simulink model "XLS_detumbling"  (R2017b)
settings: Solver=FixedStepAuto  StartTime=0.0  StopTime=25000  FixedStep=0.1  RelTol=1e-3  EnableMultiTasking=on
values from neighbouring files (symbols this model uses):
  attitude_0 = [0,0,0]    [ga_detumbling.m]    (also in ga_detumbling_fit.m = [0.0524,-0.0349,0.0175]; ga_pid.m; ga_pid_fit.m; ga_pid_test.m)
  attitude_rate_0 = [0,6.7e-05,0.0041]    [ga_detumbling.m]    (also in ga_detumbling_fit.m = [0.0873,-0.0873,-0.0873]; ga_pid.m; ga_pid_fit.m; ga_pid_test.m)
  dp = x(2)    [ga_detumbling.m]    (also in ga_detumbling_fit.m = d(2); ga_pid.m = x(4); ga_pid_fit.m = d(4); ga_pid_test.m = x(4))
  dr = x(1)    [ga_detumbling.m]    (also in ga_detumbling_fit.m = d(1); ga_pid.m = x(2); ga_pid_fit.m = d(2); ga_pid_test.m = x(2))
  dy = x(3)    [ga_detumbling.m]    (also in ga_detumbling_fit.m = d(3); ga_pid.m = x(6); ga_pid_fit.m = d(6); ga_pid_test.m = x(6))
libraries: simulink_extras x5, aerolibanim x1, sharedutil x1
CloseFcn:
  | rtwprivate ssgencode ModelCloseRequest Simul_BASE_3MW
settings Model: Creator=Kendrick  LastModifiedBy=bjt
settings SolverCC: MaxConsecutiveMinStep=5  ZeroCrossAlgorithm=Adaptive
settings DataIOCC: LimitDataPoints=on  SaveFormat=Array
settings OptimizationCC: ExpressionDepthLimit=2147483647  LifeSpan=inf
settings DebuggingCC: AlgebraicLoopMsg=none  UnderspecifiedInitializationDetection=Classic  MergeDetectMultiDrivingBlocksExec=none  SolverPrmCheckMsg=warning  FcnCallInpInsideContextMsg=warning  StateNameClashWarn=warning  SFUnexpectedBacktrackingDiag=warning  SFNoUnconditionalDefaultTransitionDiag=warning  SFExecutionAtInitializationDiag=none
settings HardwareCC: ProdBitPerInt=16  ProdBitPerPointer=16  ProdBitPerSizeT=16  ProdBitPerPtrDiffT=16  ProdLargestAtomicFloat=None  ProdIntDivRoundTo=Undefined  ProdEndianess=Unspecified  ProdWordSize=16  ProdHWDeviceType=Generic->16-bit Embedded Processor
settings ModelReferenceCC: PropagateSignalLabelsOutOfModel=off
settings CodeAppCC: StateflowObjectComments=on
settings GRTTargetCC: TargetLangStandard=C89/C90 (ANSI)  GeneratePreprocessorConditionals=Disable all  CombineOutputUpdateFcns=off  GRTInterface=on
settings ConfigComp: CovMetricSettings=dw  CovHtmlReporting=on  CovSaveCumulativeToWorkspaceVar=on  CovSaveSingleToWorkspaceVar=on  CovExternalEMLEnable=off
settings SimscapeCC: ExplicitSolverDiagnosticOptions=error  GlobalZcOffDiagnosticOptions=error  SimscapeNormalizeSystem=off
settings SimMechanicsCC: VisOnUpdateDiagram=on  VisDuringSimulation=on  LastVizWinPosition=[824 49 610 743]  CamPosition=[0.0449883;0.218364;11.4685;]  CamTarget=[-0.000193585;-0.0218554;-0.00055518;]  CamUpVector=[-0.0100593;0.999731;-0.0208998;]  CamHeight=0.706401  VisBackgroundColor=[0.9;0.9;0.95;]  DefaultBodyColor=[1;0;0;]
settings ConfigurationSet: Description=SimMechanics 2G

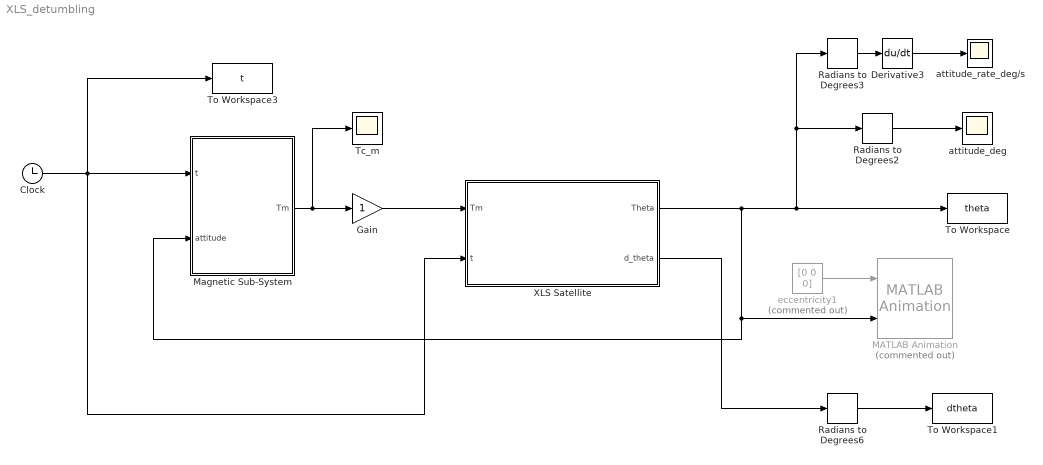
== system XLS_detumbling ==
  Clock : Clock
  Derivative3 : Derivative
  Gain : Gain
  MATLAB Animation : aerolibanim/MATLAB Animation  Tag=Matlab Animation 6 DOF  Commented=on  Vehicles=1  Geometries='XLS.mat'  BoundingBoxCoordinates=[-50,50,-50,50,-50,50]  CameraOffset=[0,0,-150]  CameraViewAngle=3  SampleTime=0.1  FigurePosition=[0,2,806,1381]
      settings: SourceProductName=Aerospace Blockset  SourceProductBaseCode=AE
  Magnetic Sub-System : Subsystem
  Radians to Degrees2 : simulink_extras/Transformations/Radians to Degrees
  Radians to Degrees3 : simulink_extras/Transformations/Radians to Degrees
  Radians to Degrees6 : simulink_extras/Transformations/Radians to Degrees
  Tc_m : Scope
  To Workspace : ToWorkspace  VariableName=theta  SampleTime=-1
  To Workspace1 : ToWorkspace  VariableName=dtheta  SampleTime=-1
  To Workspace3 : ToWorkspace  VariableName=t  SampleTime=-1
  XLS Satellite : Subsystem
  attitude_deg : Scope
  attitude_rate_deg/s : Scope
  eccentricity1 : Constant  Commented=on  Value=[0 0 0]
  wires:
  XLS Satellite/2(d_theta) -> Radians to Degrees6/1
  Gain/1 -> XLS Satellite/1(Tm)
  Derivative3/1 -> attitude_rate_deg/s/1
  Radians to Degrees2/1 -> attitude_deg/1
  Radians to Degrees3/1 -> Derivative3/1
  Magnetic Sub-System/1(Tm) -> Gain/1, Tc_m/1
  Clock/1 -> XLS Satellite/2(t), Magnetic Sub-System/1(t), To Workspace3/1
  eccentricity1/1 -> MATLAB Animation/1
  Radians to Degrees6/1 -> To Workspace1/1
  XLS Satellite/1(Theta) -> Magnetic Sub-System/2(attitude), MATLAB Animation/2, To Workspace/1, Radians to Degrees2/1, Radians to Degrees3/1

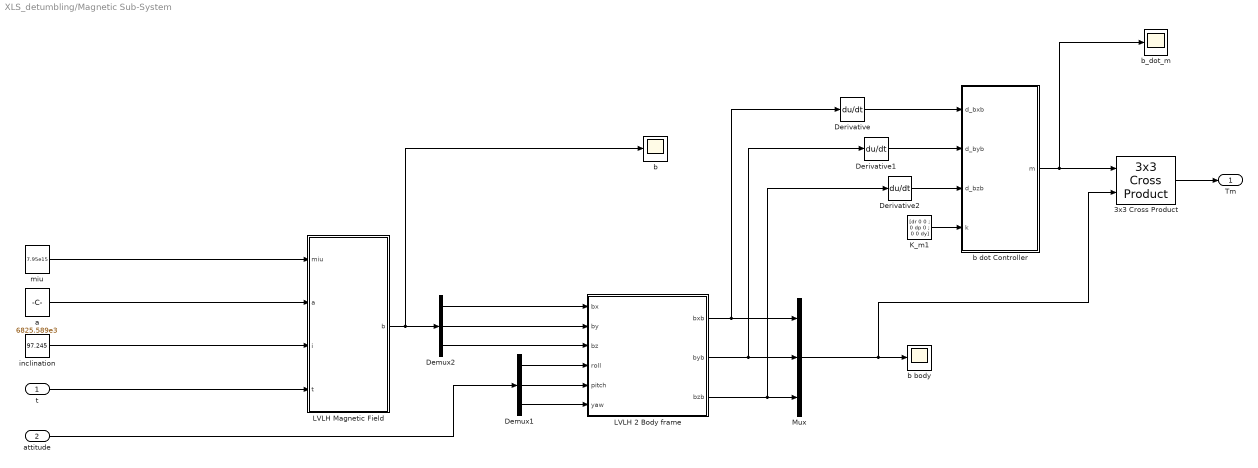
== system XLS_detumbling/Magnetic Sub-System ==
  t : Inport
  attitude : Inport  Port=2
  3x3 Cross Product : sharedutil/3x3 Cross Product
      settings: SourceProductBaseCode=AE
  Demux1 : Demux  Outputs=3
  Demux2 : Demux  Outputs=3
  Derivative : Derivative
  Derivative1 : Derivative
  Derivative2 : Derivative
  K_m1 : Constant  Value=[dr 0 0 ; 0 dp 0 ; 0 0 dy]
  LVLH 2 Body frame : MATLAB Function  TreatAsAtomicUnit=on
  LVLH Magnetic Field : MATLAB Function  TreatAsAtomicUnit=on
  Mux : Mux  Inputs=3
  a : Constant  Value=6825.589e3
  b : Scope
  b body : Scope
  b dot Controller : MATLAB Function  TreatAsAtomicUnit=on
  b_dot_m : Scope
  inclination : Constant  Value=97.245
  miu : Constant  Value=7.95e15
  Tm : Outport
  wires:
  inclination/1 -> LVLH Magnetic Field/3(i)
  t/1 -> LVLH Magnetic Field/4(t)
  Demux2/1 -> LVLH 2 Body frame/1(bx)
  Demux2/2 -> LVLH 2 Body frame/2(by)
  Demux2/3 -> LVLH 2 Body frame/3(bz)
  LVLH Magnetic Field/1(b) -> Demux2/1, b/1
  miu/1 -> LVLH Magnetic Field/1(miu)
  a/1 -> LVLH Magnetic Field/2(a)
  K_m1/1 -> b dot Controller/4(k)
  Derivative/1 -> b dot Controller/1(d_bxb)
  Derivative1/1 -> b dot Controller/2(d_byb)
  Derivative2/1 -> b dot Controller/3(d_bzb)
  Mux/1 -> 3x3 Cross Product/2, b body/1
  b dot Controller/1(m) -> b_dot_m/1, 3x3 Cross Product/1
  Demux1/1 -> LVLH 2 Body frame/4(roll)
  Demux1/2 -> LVLH 2 Body frame/5(pitch)
  Demux1/3 -> LVLH 2 Body frame/6(yaw)
  LVLH 2 Body frame/1(bxb) -> Derivative/1, Mux/1
  LVLH 2 Body frame/2(byb) -> Derivative1/1, Mux/2
  LVLH 2 Body frame/3(bzb) -> Derivative2/1, Mux/3
  3x3 Cross Product/1 -> Tm/1
  attitude/1 -> Demux1/1

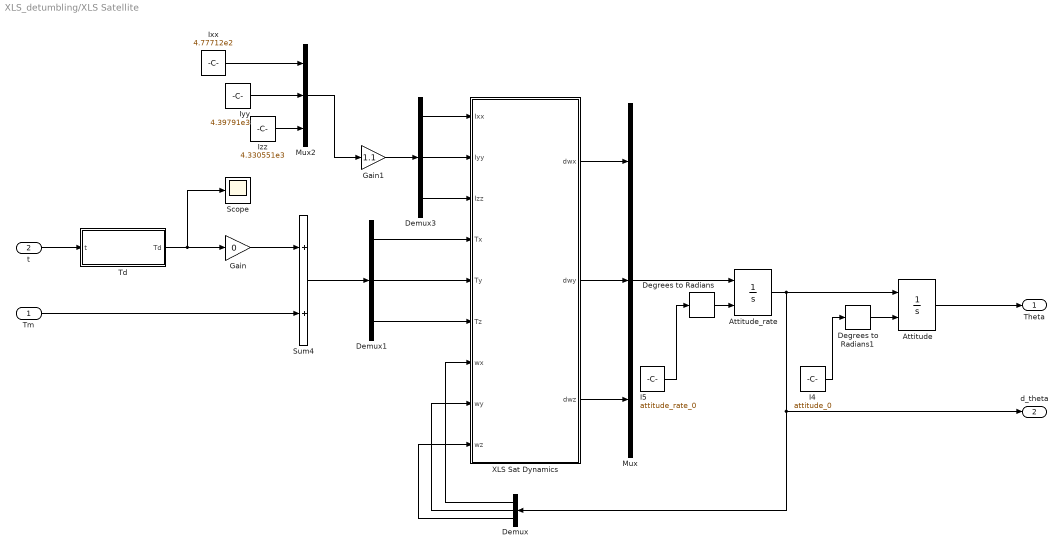
== system XLS_detumbling/XLS Satellite ==
  Tm : Inport
  t : Inport  Port=2
  Attitude : Integrator  InitialConditionSource=external
  Attitude_rate : Integrator  InitialConditionSource=external
  Degrees to Radians : simulink_extras/Transformations/Degrees to Radians
  Degrees to Radians1 : simulink_extras/Transformations/Degrees to Radians
  Demux : Demux  Outputs=3
  Demux1 : Demux  Outputs=3
  Demux3 : Demux  Outputs=3
  Gain : Gain  Gain=0
  Gain1 : Gain  Gain=1.1
  I4 : Constant  Value=attitude_0
  I5 : Constant  Value=attitude_rate_0
  Ixx : Constant  Value=4.77712e2
  Iyy : Constant  Value=4.39791e3
  Izz : Constant  Value=4.330551e3
  Mux : Mux  Inputs=3
  Mux2 : Mux  Inputs=3
  Scope : Scope
  Sum4 : Sum
  Td : Subsystem
  XLS Sat Dynamics : MATLAB Function  TreatAsAtomicUnit=on
  Theta : Outport
  d_theta : Outport  Port=2
  wires:
  t/1 -> Td/1(t)
  Attitude/1 -> Theta/1
  Attitude_rate/1 -> Attitude/1, Demux/1, d_theta/1
  Demux/1 -> XLS Sat Dynamics/7(wx)
  Demux/2 -> XLS Sat Dynamics/8(wy)
  Demux/3 -> XLS Sat Dynamics/9(wz)
  XLS Sat Dynamics/1(dwx) -> Mux/1
  XLS Sat Dynamics/2(dwy) -> Mux/2
  XLS Sat Dynamics/3(dwz) -> Mux/3
  Mux/1 -> Attitude_rate/1
  Td/1(Td) -> Scope/1, Gain/1
  Tm/1 -> Sum4/2
  I4/1 -> Degrees to Radians1/1
  I5/1 -> Degrees to Radians/1
  Degrees to Radians/1 -> Attitude_rate/2
  Degrees to Radians1/1 -> Attitude/2
  Sum4/1 -> Demux1/1
  Gain/1 -> Sum4/1
  Demux1/1 -> XLS Sat Dynamics/4(Tx)
  Demux1/2 -> XLS Sat Dynamics/5(Ty)
  Demux3/3 -> XLS Sat Dynamics/3(Izz)
  Demux3/2 -> XLS Sat Dynamics/2(Iyy)
  Demux3/1 -> XLS Sat Dynamics/1(Ixx)
  Gain1/1 -> Demux3/1
  Mux2/1 -> Gain1/1
  Ixx/1 -> Mux2/1
  Izz/1 -> Mux2/3
  Iyy/1 -> Mux2/2
  Demux1/3 -> XLS Sat Dynamics/6(Tz)

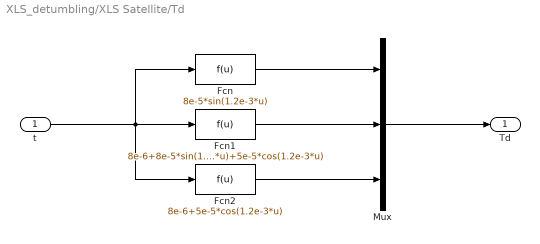
== system XLS_detumbling/XLS Satellite/Td ==
  t : Inport
  Fcn : Fcn  Expr=8e-5*sin(1.2e-3*u)
  Fcn1 : Fcn  Expr=8e-6+8e-5*sin(1.2e-3*u)+5e-5*cos(1.2e-3*u)
  Fcn2 : Fcn  Expr=8e-6+5e-5*cos(1.2e-3*u)
  Mux : Mux  Inputs=3
  Td : Outport
  wires:
  t/1 -> Fcn1/1, Fcn/1, Fcn2/1
  Fcn1/1 -> Mux/2
  Fcn/1 -> Mux/1
  Fcn2/1 -> Mux/3
  Mux/1 -> Td/1

== matlab function XLS_detumbling/XLS Satellite/XLS Sat Dynamics ==
  data: Ixx input; Iyy input; Izz input; Tx input; Ty input; Tz input; wx input; wy input; wz input; dwx output; dwy output; dwz output
function [dwx,dwy,dwz] = Satellite(Ixx,Iyy,Izz,Tx,Ty,Tz,wx,wy,wz)

dwx = (Tx-(Iyy-Izz)*wz*wy)/Ixx;
dwy = (Ty-(Izz-Ixx)*wx*wz)/Iyy;
dwz = (Tz-(Ixx-Iyy)*wy*wx)/Izz;

== matlab function XLS_detumbling/Magnetic Sub-System/LVLH 2 Body frame ==
  data: bx input; bxb output; by input; bz input; roll input; pitch input; yaw input; byb output; bzb output
function [bxb,byb,bzb] = fcn(bx,by,bz,roll,pitch,yaw)
bb=[cos(pitch)          ,-cos(yaw)*sin(pitch)                               ,sin(pitch)*sin(yaw);
    cos(roll)*sin(pitch), cos(roll)*cos(pitch)*cos(yaw)-sin(roll)*sin(yaw)  ,-cos(yaw)*sin(roll)-cos(roll)*cos(pitch)*sin(yaw);
    sin(roll)*sin(pitch), cos(roll)*sin(yaw)+cos(pitch)*cos(yaw)*sin(roll)   , cos(roll)*cos(yaw)-cos(pitch)*sin(roll)*sin(yaw)]*[bx;by;bz];
bxb=bb(1);
byb=bb(2);
bzb=bb(3);

== matlab function XLS_detumbling/Magnetic Sub-System/LVLH Magnetic Field ==
  data: miu input; a input; i input; b output; t input
function b = magnetic_field(miu,a,i,t)

b = miu/a^3*[sin(deg2rad(i))*cos(1.2e-3*t);
    -cos(deg2rad(i));
    2*sin(deg2rad(i))*sin(1.2e-3*t)];

== matlab function XLS_detumbling/Magnetic Sub-System/b dot Controller ==
  data: d_bxb input; d_byb input; d_bzb input; k input; m output
function m = fcn(d_bxb, d_byb, d_bzb, k)
m=-k*[d_bxb ;d_byb ;d_bzb];
for i=1:3
    if m(i)>110
        m(i)=110;
    end
    if m(i)<-110
        m(i)=-110;
    end
end
%cross(m,[bxb ; byb ; bzb]);
